simulink model "two_dof_arm_with_lqr_with_simscape"  (R2023a)
settings: Solver=FixedStepAuto  StartTime=0.0  StopTime=5  FixedStep=0.001  RelTol=1e-3
InitFcn:
  | two_link_planar_manipulator_sim
values from neighbouring files (symbols this model uses):
  g = [0 -9.81 0]    [two_link_planar_manipulator_sim.m]
  K = lqr(A,B,Q,R)    [two_link_planar_manipulator_sim.m]
  l = [0.25 0.25]    [two_link_planar_manipulator_sim.m]
  m = [1 1]    [two_link_planar_manipulator_sim.m]
  offset_error = 0.0175    [two_link_planar_manipulator_sim.m]
  resolution = 2^12    (= 4096)    [two_link_planar_manipulator_sim.m]
  sample_time = 0.001    [two_link_planar_manipulator_sim.m]
  true_delay = floor(delay*10^-3/sample_time)+sample_time*10^3    [two_link_planar_manipulator_sim.m]
  w = [0.04 0.04]    [two_link_planar_manipulator_sim.m]
  without_actuator_dynamics = true    [two_link_planar_manipulator_sim.m]
  without_meas_uncertainty = false    [two_link_planar_manipulator_sim.m]
libraries: sm_lib x12, nesl_utility x7, spsFirstOrderFilterLib x2, simulink x2, robotmaniplib x1, robotcorelib x1
settings Model: Creator=Jordan  LastModifiedBy=ddominguezmoises

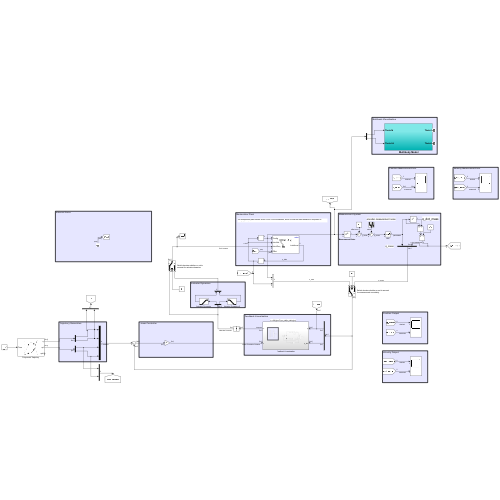
[thumbnail: Simulink's stored preview of the top-level diagram]
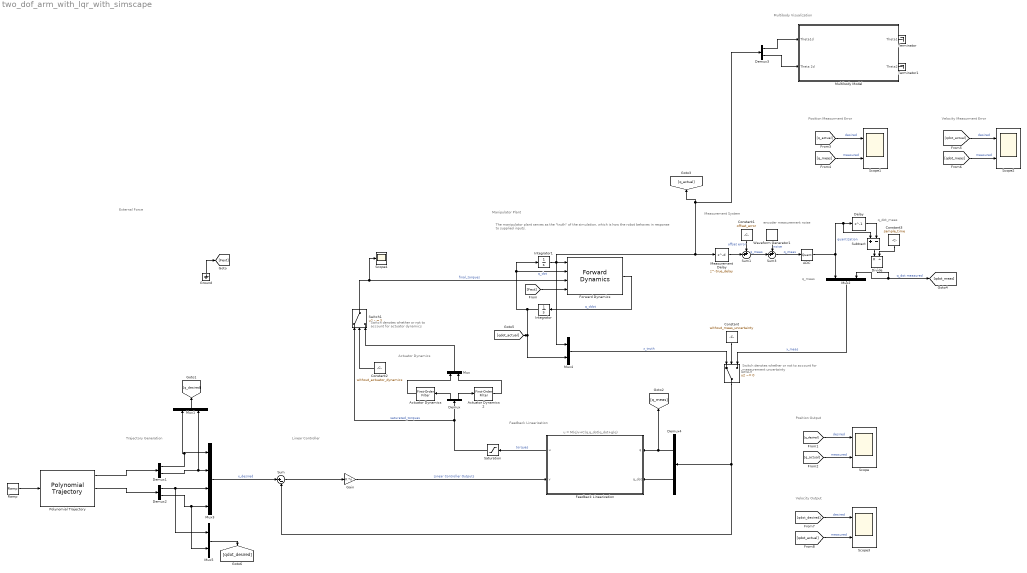
== system two_dof_arm_with_lqr_with_simscape ==
  note: Position Output
  note: Actuator Dynamics
  note: Switch denotes whether or not to account for actuator dynamics
  note: Switch denotes whether or not to account for measurement uncertainty
  note: u = M(q)v+C(q,q_dot)q_dot+g(q)
  note: Manipulator Plant
  note: The manipulator plant serves as the "truth" of the simulation, which is how the robot behaves in response to supplied inputs.
  note: Trajectory Generation
  note: Linear Controller
  note: Measurement System
  note: q_dot_meas
  note: encoder measurement noise
  note: q_meas
  note: Feedback Linearization
  note: External Force
  note: Position Measurment Error
  note: Velocity Measurment Error
  note: Velocity Output
  note: Multibody Visualization
  " Multibody Model" : Subsystem
  ADC : Quantizer  QuantizationInterval=2*pi/resolution  LinearizeAsGain=off
  Actuator Dynamics : spsFirstOrderFilterLib/First-Order Filter  FilterType=Lowpass  Tc=4.389e-4  Ts=0  Initialize=off  Vac_Init=[0, 0, 60]  Vdc_Init=0  PlotResponse=off  FreqRange="[0,  200,  1]"
  Actuator Dynamics 2 : spsFirstOrderFilterLib/First-Order Filter  FilterType=Lowpass  Tc=4.389e-4  Ts=0  Initialize=off  Vac_Init=[0, 0, 60]  Vdc_Init=0  PlotResponse=off  FreqRange="[0,  200,  1]"
  Constant : Constant  Value=without_meas_uncertainty
  Constant1 : Constant  Value=offset_error
  Constant2 : Constant  Value=without_actuator_dynamics
  Constant3 : Constant  Value=sample_time
  Delay : Delay  DelayLength=1
  Demux{,1..4} (5 alike) : Demux  Outputs=2
  Divide : Product  Inputs=*/
  Feedback Linearization : Subsystem
      settings: PortSchema="{\"entries\":[{\"content\":{\"sides\":[{\"content\":{\"connectorIds\":[\"In1\",\"In2\"]},\"type\":\"ConnectorPlacement.EquallySpacedRectSide\",\"uuid\":\"e20634ac-7282-4506-b427-a1989d27ee42\"},{\"content\":{\"connectorIds\":[\"Out1\",\"In3\"],\"side\":\"RIGHT\"},\"type\":\"ConnectorPlacement.EquallySpacedRectSide\",\"uuid\":\"ff8f2b23-ed86-4124-b979-83474755293e\"},{\"content\":{\"side\":\"TOP\"},\"type\":\"ConnectorPlacement.EquallySpacedRectSide\",\"uuid\":\"75dc970f-ba8d-4ce0-9b15-e79bd05d50ba\"}]},\"type\":\"ConnectorPlacement.EquallySpacedConnector\",\"uuid\":\"cd5a2392-675b-4624-9569-e6445bfb2136\"}],\"packageUris\":[\"http://schema.mathworks.com/mf0/Connector/R2020b\"],\"version\":\"1.0\"}"
  Forward Dynamics : robotmaniplib/Forward Dynamics  RigidBodyTree=robot  SimulateUsing=Interpreted execution
  Gain : Gain  Gain=K  Multiplication=Matrix(K*u)
  Ground : Ground
  Integrator : Integrator  InitialCondition=[0;0]
  Integrator1 : Integrator  InitialCondition=[0;0]
  Measurement Delay : Delay  DelayLength=true_delay
  Mux{,1..2,4..5} (5 alike) : Mux  Inputs=2
  Mux3 : Mux
  Polynomial Trajectory : robotcorelib/Polynomial Trajectory  WaypointSource=Internal  Waypoints=[ 0, 0, pi/2; 0, 0, pi/2]  TimePoints=[ 0, 1, 1.5]  TimeInterval=[ 1, 4 ]  Method=Cubic Polynomial  ParameterSource=Internal  VelocityBoundaryCondition=zeros( 2, 3 )  AccelerationBoundaryCondition=zeros( 2, 3 )  SimulateUsing=Interpreted execution
  Ramp : simulink/Sources/Ramp  slope=1  start=0  InitialOutput=0
  Saturation : Saturate  UpperLimit=150  LowerLimit=-150
  Scope{,1..3} (4 alike) : Scope  NumInputPorts=2
  Scope4 : Scope
  Subtract : Sum  Inputs=+-
  Sum : Sum  Inputs=|+-
  Sum1 : Sum  Inputs=++|
  Sum3 : Sum  Inputs=++|
  Switch : Switch  Criteria=u2 ~= 0  SaturateOnIntegerOverflow=off  InputSameDT=off
  Switch1 : Switch  Criteria=u2 ~= 0  SaturateOnIntegerOverflow=off  InputSameDT=off
  Terminator : Terminator
  Terminator1 : Terminator
  Waveform Generator1 : simulink/Sources/Waveform Generator  OutMin=[]  OutMax=[]  OutDataTypeStr=double  SelectedSignal=1  Signals=gaussian(mean,variance, seed)#gaussian(mean,variance, seed)  BlockNames=MultiportSwitch_510e73f99105412#MultiportSwitch_1249e3761ae8455  SampleTime=0.1
  wires:
  Integrator/1 -> [qdot_actual], Mux4/2, Integrator1/1, Forward Dynamics/2  "q_dot"
  Forward Dynamics/1 -> Integrator/1  "q_ddot"
  Delay/1 -> Subtract/2
  Sum3/1 -> ADC/1  "q_meas"
  Waveform Generator1/1 -> Sum3/1  "noise"
  Feedback Linearization/1(u) -> Saturation/1  "torques"
  Demux4/1 -> Feedback Linearization/1(q), [q_meas]
  Demux4/2 -> Feedback Linearization/2(q_dot)
  Gain/1 -> Feedback Linearization/3(v)  "Linear Controller Outputs"
  Ground/1 -> [Fext]
  [Fext] -> Forward Dynamics/4
  Sum1/1 -> Sum3/2  "q_meas"
  Constant1/1 -> Sum1/1  "offset error"
  Measurement Delay/1 -> Sum1/2
  ADC/1 -> Subtract/1, Delay/1, Mux2/1  "quantization"
  Demux/2 -> Actuator Dynamics 2/1
  Demux/1 -> Actuator Dynamics/1
  Actuator Dynamics/1 -> Mux/1
  Actuator Dynamics 2/1 -> Mux/2
  Mux1/1 -> [q_desired]
  Mux3/1 -> Sum/1  "x_desired"
  Sum/1 -> Gain/1
  Mux4/1 -> Switch/1  "x_truth"
  Mux2/1 -> Switch/3  "x_meas"
  Constant/1 -> Switch/2
  Switch/1 -> Demux4/1, Sum/2
  Switch1/1 -> Scope4/1, Forward Dynamics/3  "final_torques"
  Constant2/1 -> Switch1/2
  [q_desired] -> Scope/1  "desired"
  [q_actual] -> Scope/2  "measured"
  [q_actual] -> Scope1/1  "desired"
  [q_meas] -> Scope1/2  "measured"
  Subtract/1 -> Divide/1
  Constant3/1 -> Divide/2
  Divide/1 -> [qdot_meas], Mux2/2  "q_dot measured"
  [qdot_meas] -> Scope2/2  "measured"
  [qdot_actual] -> Scope2/1  "desired"
  [qdot_actual] -> Scope3/2  "measured"
  [qdot_desired] -> Scope3/1  "desired"
  Mux5/1 -> [qdot_desired]
  Mux/1 -> Switch1/3
  Ramp/1 -> Polynomial Trajectory/1
  Polynomial Trajectory/1 -> Demux1/1
  Demux1/1 -> Mux1/1, Mux3/1
  Demux1/2 -> Mux1/2, Mux3/2
  Polynomial Trajectory/2 -> Demux2/1
  Demux2/1 -> Mux5/1, Mux3/3
  Demux2/2 -> Mux5/2, Mux3/4
  Saturation/1 -> Demux/1, Switch1/1  "saturated_torques"
  " Multibody Model"/1(Theta1) -> Terminator/1
  " Multibody Model"/2(Theta2) -> Terminator1/1
  Demux3/2 -> " Multibody Model"/2(Theta 2d)
  Demux3/1 -> " Multibody Model"/1(Theta1d)
  Integrator1/1 -> Forward Dynamics/1, Mux4/1, Measurement Delay/1, Demux3/1, [q_actual]

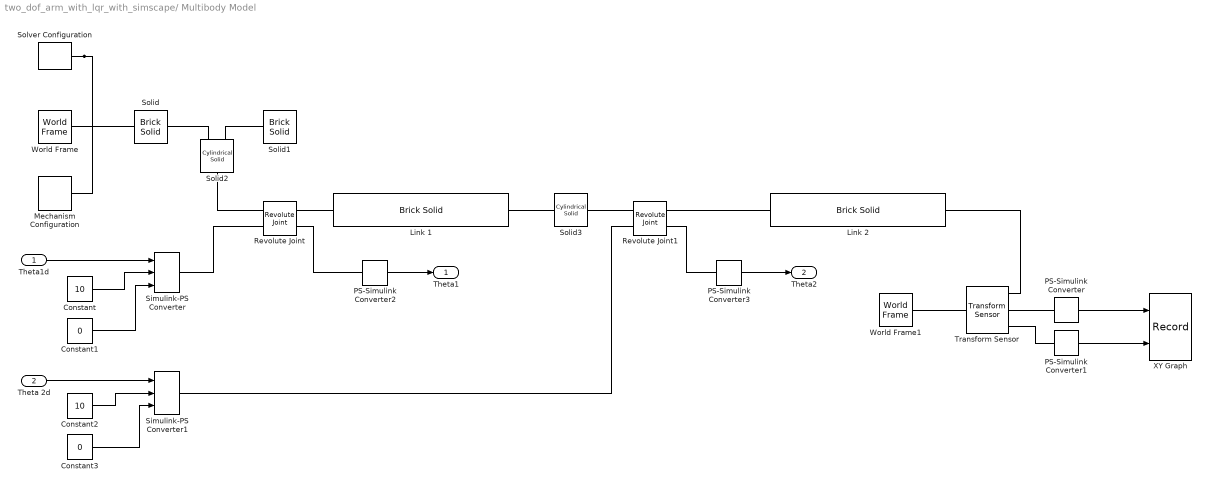
== system two_dof_arm_with_lqr_with_simscape/ Multibody Model ==
  Theta1d : Inport
  Theta 2d : Inport  Port=2
  Constant : Constant  Value=10
  Constant1 : Constant  Value=0
  Constant2 : Constant  Value=10
  Constant3 : Constant  Value=0
  Link 1 : sm_lib/Body Elements/Brick Solid  GraphicAmbientColor=[0.15 0.15 0.15 1.0]  BasedOnType=Density  BrickDimensions=[100 15 5]  BrickDimensionsUnits=cm  CenterOfMass=[0 0 0]  CenterOfMassUnits=m  GraphicDiffuseColor=[1.0 0.4 0.4]  Density=1000  DensityUnits=kg/m^3  DoExposeReferenceFrame=off  GraphicEmissiveColor=[0.0 0.0 0.0 1.0]  ExportEntireGeometry=off  SerializedFrames=<Frames><Frame><Id>Frame1</Id><Value><Name>L</Name><Origin><Source>GeometricFeature</Source><FeatureName>-x surface</FeatureName></Origin><PrimaryAxis><DefinedDirection>+Z</DefinedDirection><Source>ReferenceFrame</Source><SourceDirection>+Z</SourceDirection><FeatureName></FeatureName></PrimaryAxis><SecondaryAxis><DefinedDirection>+X</DefinedDirection><Source>ReferenceFrame</Source><SourceDirection>+X</SourceDirection><FeatureName></FeatureName></SecondaryAxis></Value></Frame><Frame><Id>Frame2</Id><Value><Name>R</Name><Origin><Source>GeometricFeature</Source><FeatureName>+x surface</FeatureName></Origin><PrimaryAxis><DefinedDirection>+Z</DefinedDirection><Source>ReferenceFrame</Source><SourceDirection>+Z</SourceDirection><FeatureName></FeatureName></PrimaryAxis><SecondaryAxis><DefinedDirection>+X</DefinedDirection><Source>ReferenceFrame</Source><SourceDirection>+X</SourceDirection><FeatureName></FeatureName></SecondaryAxis></Value></Frame></Frames>  MarkerShape=Sphere  MarkerSize=10  GraphicType=FromGeometry  InertiaType=CalculateFromGeometry  Mass=1  MassUnits=kg  MomentsOfInertia=[1 1 1]  MomentsOfInertiaUnits=kg*m^2  GraphicOpacity=1.0  ProductsOfInertia=[1 1 1]  ProductsOfInertiaUnits=kg*m^2  GraphicShininess=75  GraphicSpecularColor=[0.5 0.5 0.5 1.0]  GraphicVisPropType=SimpleVisualProperties
  Link 2 : sm_lib/Body Elements/Brick Solid  GraphicAmbientColor=[0.15 0.15 0.15 1.0]  BasedOnType=Density  BrickDimensions=[100 15 5]  BrickDimensionsUnits=cm  CenterOfMass=[0 0 0]  CenterOfMassUnits=m  GraphicDiffuseColor=[0.0 0.4 0.0]  Density=1000  DensityUnits=kg/m^3  DoExposeReferenceFrame=off  GraphicEmissiveColor=[0.0 0.0 0.0 1.0]  ExportEntireGeometry=off  SerializedFrames=<Frames><Frame><Id>Frame1</Id><Value><Name>L</Name><Origin><Source>GeometricFeature</Source><FeatureName>-x surface</FeatureName></Origin><PrimaryAxis><DefinedDirection>+Z</DefinedDirection><Source>ReferenceFrame</Source><SourceDirection>+Z</SourceDirection><FeatureName></FeatureName></PrimaryAxis><SecondaryAxis><DefinedDirection>+X</DefinedDirection><Source>ReferenceFrame</Source><SourceDirection>+X</SourceDirection><FeatureName></FeatureName></SecondaryAxis></Value></Frame><Frame><Id>Frame2</Id><Value><Name>R</Name><Origin><Source>GeometricFeature</Source><FeatureName>+x surface</FeatureName></Origin><PrimaryAxis><DefinedDirection>+Z</DefinedDirection><Source>ReferenceFrame</Source><SourceDirection>+Z</SourceDirection><FeatureName></FeatureName></PrimaryAxis><SecondaryAxis><DefinedDirection>+X</DefinedDirection><Source>ReferenceFrame</Source><SourceDirection>+X</SourceDirection><FeatureName></FeatureName></SecondaryAxis></Value></Frame></Frames>  MarkerShape=Sphere  MarkerSize=10  GraphicType=FromGeometry  InertiaType=CalculateFromGeometry  Mass=1  MassUnits=kg  MomentsOfInertia=[1 1 1]  MomentsOfInertiaUnits=kg*m^2  GraphicOpacity=1.0  ProductsOfInertia=[1 1 1]  ProductsOfInertiaUnits=kg*m^2  GraphicShininess=75  GraphicSpecularColor=[0.5 0.5 0.5 1.0]  GraphicVisPropType=SimpleVisualProperties
  Mechanism Configuration : sm_lib/Utilities/Mechanism Configuration  UniformGravity=Constant  GravityVector=[0 -9.80665 0]  GravityVectorUnits=m/s^2  LinearizationDelta=0.001  JointModeTransitionNonlinearIterations=2
  PS-Simulink Converter{,1..3} (4 alike) : nesl_utility/PS-Simulink Converter  PhysicalDomain=network_engine_domain  SubClassName=ps_output  LeftPortType=input  RightPortType=output  PseudoPeriodic=off  Frequencies=[]  VectorFormat=1-D array  Unit=1  AffineConversion=off
  Revolute Joint : sm_lib/Joints/Revolute Joint  JointMode=Normal  SenseConstraintForce=off  SenseConstraintForceX=off  SenseConstraintForceY=off  SenseConstraintForceZ=off  SenseConstraintTorque=off  SenseConstraintTorqueX=off  SenseConstraintTorqueY=off  SenseConstraintTorqueZ=off  SenseTotalForce=off  SenseTotalForceX=off  SenseTotalForceY=off  SenseTotalForceZ=off  SenseTotalTorque=off  SenseTotalTorqueX=off  SenseTotalTorqueY=off  SenseTotalTorqueZ=off  CompositeWrenchDir=FollowerOnBase  CompositeWrenchFrame=BaseFrame  EquilibriumPosition=0  EquilibriumPositionUnits=deg  SpringStiffness=0  SpringStiffnessUnits=N*m/deg  DampingCoefficient=0  DampingCoefficientUnits=N*m/(deg/s)  TorqueActuationMode=ComputedTorque  MotionActuationMode=InputMotion  SensePosition=on  SenseVelocity=off  SenseAcceleration=off  SenseTorqueForce=off  SenseLowerLimitTorqueForce=off  SenseUpperLimitTorqueForce=off  LowerLimitSpecify=off  LowerLimitBound=-90  LowerLimitBoundUnits=deg  LowerLimitStiffness=1e4  LowerLimitStiffnessUnits=N*m/deg  LowerLimitDamping=10  LowerLimitDampingUnits=N*m/(deg/s)  LowerLimitTransitionRegionWidth=0.1  LowerLimitTransitionRegionWidthUnits=deg  UpperLimitSpecify=off  UpperLimitBound=90  UpperLimitBoundUnits=deg  UpperLimitStiffness=1e4  UpperLimitStiffnessUnits=N*m/deg  UpperLimitDamping=10  UpperLimitDampingUnits=N*m/(deg/s)  UpperLimitTransitionRegionWidth=0.1  UpperLimitTransitionRegionWidthUnits=deg  PositionTargetSpecify=off  PositionTargetPriority=High  PositionTargetValue=0  PositionTargetValueUnits=deg  VelocityTargetSpecify=off  VelocityTargetPriority=High  VelocityTargetValue=0  VelocityTargetValueUnits=deg/s
  Revolute Joint1 : sm_lib/Joints/Revolute Joint  JointMode=Normal  SenseConstraintForce=off  SenseConstraintForceX=off  SenseConstraintForceY=off  SenseConstraintForceZ=off  SenseConstraintTorque=off  SenseConstraintTorqueX=off  SenseConstraintTorqueY=off  SenseConstraintTorqueZ=off  SenseTotalForce=off  SenseTotalForceX=off  SenseTotalForceY=off  SenseTotalForceZ=off  SenseTotalTorque=off  SenseTotalTorqueX=off  SenseTotalTorqueY=off  SenseTotalTorqueZ=off  CompositeWrenchDir=FollowerOnBase  CompositeWrenchFrame=BaseFrame  EquilibriumPosition=0  EquilibriumPositionUnits=deg  SpringStiffness=0  SpringStiffnessUnits=N*m/deg  DampingCoefficient=0  DampingCoefficientUnits=N*m/(deg/s)  TorqueActuationMode=ComputedTorque  MotionActuationMode=InputMotion  SensePosition=on  SenseVelocity=off  SenseAcceleration=off  SenseTorqueForce=off  SenseLowerLimitTorqueForce=off  SenseUpperLimitTorqueForce=off  LowerLimitSpecify=off  LowerLimitBound=-90  LowerLimitBoundUnits=deg  LowerLimitStiffness=1e4  LowerLimitStiffnessUnits=N*m/deg  LowerLimitDamping=10  LowerLimitDampingUnits=N*m/(deg/s)  LowerLimitTransitionRegionWidth=0.1  LowerLimitTransitionRegionWidthUnits=deg  UpperLimitSpecify=off  UpperLimitBound=90  UpperLimitBoundUnits=deg  UpperLimitStiffness=1e4  UpperLimitStiffnessUnits=N*m/deg  UpperLimitDamping=10  UpperLimitDampingUnits=N*m/(deg/s)  UpperLimitTransitionRegionWidth=0.1  UpperLimitTransitionRegionWidthUnits=deg  PositionTargetSpecify=off  PositionTargetPriority=High  PositionTargetValue=0  PositionTargetValueUnits=deg  VelocityTargetSpecify=off  VelocityTargetPriority=High  VelocityTargetValue=0  VelocityTargetValueUnits=deg/s
  Simulink-PS Converter : nesl_utility/Simulink-PS Converter  PhysicalDomain=network_engine_domain  SubClassName=ps_input  LeftPortType=input  RightPortType=output  PseudoPeriodic=off  Frequencies=[]  NoiseDistribution=none  NoiseParameters=[]  Unit=1  AffineConversion=off  FilteringAndDerivatives=provide  SimscapeFilterOrder=1  InputFilterTimeConstant=0.001  UdotUserProvided=2
  Simulink-PS Converter1 : nesl_utility/Simulink-PS Converter  PhysicalDomain=network_engine_domain  SubClassName=ps_input  LeftPortType=input  RightPortType=output  PseudoPeriodic=off  Frequencies=[]  NoiseDistribution=none  NoiseParameters=[]  Unit=1  AffineConversion=off  FilteringAndDerivatives=provide  SimscapeFilterOrder=1  InputFilterTimeConstant=0.001  UdotUserProvided=2
  Solid : sm_lib/Body Elements/Brick Solid  GraphicAmbientColor=[0.15 0.15 0.15 1.0]  BasedOnType=Density  BrickDimensions=[15 15 5]  BrickDimensionsUnits=cm  CenterOfMass=[0 0 0]  CenterOfMassUnits=m  GraphicDiffuseColor=[0.0 0.0 0.6]  Density=1000  DensityUnits=kg/m^3  DoExposeReferenceFrame=on  GraphicEmissiveColor=[0.0 0.0 0.0 1.0]  ExportEntireGeometry=off  SerializedFrames=<Frames><Frame><Id>Frame1</Id><Value><Name>F</Name><Origin><Source>GeometricFeature</Source><FeatureName>-z surface</FeatureName></Origin><PrimaryAxis><DefinedDirection>+Z</DefinedDirection><Source>ReferenceFrame</Source><SourceDirection>+Z</SourceDirection><FeatureName></FeatureName></PrimaryAxis><SecondaryAxis><DefinedDirection>+X</DefinedDirection><Source>ReferenceFrame</Source><SourceDirection>+X</SourceDirection><FeatureName></FeatureName></SecondaryAxis></Value></Frame></Frames>  MarkerShape=Sphere  MarkerSize=10  GraphicType=FromGeometry  InertiaType=CalculateFromGeometry  Mass=1  MassUnits=kg  MomentsOfInertia=[1 1 1]  MomentsOfInertiaUnits=kg*m^2  GraphicOpacity=1.0  ProductsOfInertia=[1 1 1]  ProductsOfInertiaUnits=kg*m^2  GraphicShininess=75  GraphicSpecularColor=[0.5 0.5 0.5 1.0]  GraphicVisPropType=SimpleVisualProperties
  Solid1 : sm_lib/Body Elements/Brick Solid  GraphicAmbientColor=[0.15 0.15 0.15 1.0]  BasedOnType=Density  BrickDimensions=[15 15 5]  BrickDimensionsUnits=cm  CenterOfMass=[0 0 0]  CenterOfMassUnits=m  GraphicDiffuseColor=[0.0 0.0 0.6]  Density=1000  DensityUnits=kg/m^3  DoExposeReferenceFrame=off  GraphicEmissiveColor=[0.0 0.0 0.0 1.0]  ExportEntireGeometry=off  SerializedFrames=<Frames><Frame><Id>Frame1</Id><Value><Name>F</Name><Origin><Source>GeometricFeature</Source><FeatureName>+z surface</FeatureName></Origin><PrimaryAxis><DefinedDirection>+Z</DefinedDirection><Source>ReferenceFrame</Source><SourceDirection>+Z</SourceDirection><FeatureName></FeatureName></PrimaryAxis><SecondaryAxis><DefinedDirection>+X</DefinedDirection><Source>ReferenceFrame</Source><SourceDirection>+X</SourceDirection><FeatureName></FeatureName></SecondaryAxis></Value></Frame></Frames>  MarkerShape=Sphere  MarkerSize=10  GraphicType=FromGeometry  InertiaType=CalculateFromGeometry  Mass=1  MassUnits=kg  MomentsOfInertia=[1 1 1]  MomentsOfInertiaUnits=kg*m^2  GraphicOpacity=1.0  ProductsOfInertia=[1 1 1]  ProductsOfInertiaUnits=kg*m^2  GraphicShininess=75  GraphicSpecularColor=[0.5 0.5 0.5 1.0]  GraphicVisPropType=SimpleVisualProperties
  Solid2 : sm_lib/Body Elements/Cylindrical Solid  GraphicAmbientColor=[0.15 0.15 0.15 1.0]  BasedOnType=Density  CenterOfMass=[0 0 0]  CenterOfMassUnits=m  GraphicDiffuseColor=[0.0 0.0 0.6]  CylinderLength=6  CylinderLengthUnits=cm  CylinderRadius=5  CylinderRadiusUnits=cm  Density=1000  DensityUnits=kg/m^3  DoExposeReferenceFrame=on  GraphicEmissiveColor=[0.0 0.0 0.0 1.0]  ExportEntireGeometry=off  SerializedFrames=<Frames><Frame><Id>Frame1</Id><Value><Name>L</Name><Origin><Source>GeometricFeature</Source><FeatureName>top surface</FeatureName></Origin><PrimaryAxis><DefinedDirection>+Z</DefinedDirection><Source>ReferenceFrame</Source><SourceDirection>+Z</SourceDirection><FeatureName></FeatureName></PrimaryAxis><SecondaryAxis><DefinedDirection>+X</DefinedDirection><Source>ReferenceFrame</Source><SourceDirection>+X</SourceDirection><FeatureName></FeatureName></SecondaryAxis></Value></Frame><Frame><Id>Frame2</Id><Value><Name>R</Name><Origin><Source>GeometricFeature</Source><FeatureName>bottom surface</FeatureName></Origin><PrimaryAxis><DefinedDirection>+Z</DefinedDirection><Source>ReferenceFrame</Source><SourceDirection>+Z</SourceDirection><FeatureName></FeatureName></PrimaryAxis><SecondaryAxis><DefinedDirection>+X</DefinedDirection><Source>ReferenceFrame</Source><SourceDirection>+X</SourceDirection><FeatureName></FeatureName></SecondaryAxis></Value></Frame></Frames>  MarkerShape=Sphere  MarkerSize=10  GraphicType=FromGeometry  InertiaType=CalculateFromGeometry  Mass=1  MassUnits=kg  MomentsOfInertia=[1 1 1]  MomentsOfInertiaUnits=kg*m^2  GraphicOpacity=1.0  ProductsOfInertia=[1 1 1]  ProductsOfInertiaUnits=kg*m^2  GraphicShininess=75  GraphicSpecularColor=[0.5 0.5 0.5 1.0]  GraphicVisPropType=SimpleVisualProperties
  Solid3 : sm_lib/Body Elements/Cylindrical Solid  GraphicAmbientColor=[0.15 0.15 0.15 1.0]  BasedOnType=Density  CenterOfMass=[0 0 0]  CenterOfMassUnits=m  GraphicDiffuseColor=[0.8 0.0 0.0]  CylinderLength=6  CylinderLengthUnits=cm  CylinderRadius=5  CylinderRadiusUnits=cm  Density=1000  DensityUnits=kg/m^3  DoExposeReferenceFrame=off  GraphicEmissiveColor=[0.0 0.0 0.0 1.0]  ExportEntireGeometry=off  SerializedFrames=<Frames><Frame><Id>Frame1</Id><Value><Name>L</Name><Origin><Source>GeometricFeature</Source><FeatureName>top surface</FeatureName></Origin><PrimaryAxis><DefinedDirection>+Z</DefinedDirection><Source>ReferenceFrame</Source><SourceDirection>+Z</SourceDirection><FeatureName></FeatureName></PrimaryAxis><SecondaryAxis><DefinedDirection>+X</DefinedDirection><Source>ReferenceFrame</Source><SourceDirection>+X</SourceDirection><FeatureName></FeatureName></SecondaryAxis></Value></Frame><Frame><Id>Frame2</Id><Value><Name>R</Name><Origin><Source>GeometricFeature</Source><FeatureName>bottom surface</FeatureName></Origin><PrimaryAxis><DefinedDirection>+Z</DefinedDirection><Source>ReferenceFrame</Source><SourceDirection>+Z</SourceDirection><FeatureName></FeatureName></PrimaryAxis><SecondaryAxis><DefinedDirection>+X</DefinedDirection><Source>ReferenceFrame</Source><SourceDirection>+X</SourceDirection><FeatureName></FeatureName></SecondaryAxis></Value></Frame></Frames>  MarkerShape=Sphere  MarkerSize=10  GraphicType=FromGeometry  InertiaType=CalculateFromGeometry  Mass=1  MassUnits=kg  MomentsOfInertia=[1 1 1]  MomentsOfInertiaUnits=kg*m^2  GraphicOpacity=1.0  ProductsOfInertia=[1 1 1]  ProductsOfInertiaUnits=kg*m^2  GraphicShininess=75  GraphicSpecularColor=[0.5 0.5 0.5 1.0]  GraphicVisPropType=SimpleVisualProperties
  Solver Configuration : nesl_utility/Solver Configuration  PhysicalDomain=network_engine_domain  SubClassName=solver  LeftPortType=input  RightPortType=generic  Tones=[]  Harmonics=[]  SimulateNoise=off  Profile=off  UseLocalSampling=off  EnableSwitchedLinearOptims=on  FrequencyDomain=off  UseCCode=off  RelTol=0.001  AbsTol=1e-06  MinStep=1e-09  ToWorkspace=off  RevertToSquareIcSolve=off  NumHomotopyIterations=100  PhasorMode=off  PhasorModeNumHarmonics=1  ConsistencySolver=NEWTON_FTOL  IndexReductionMethod=DerivativeReplacement  DoDC=off  ResidualTolerance=1e-09  ConsistencyTolSource=GLOBAL  ConsistencyAbsTol=0.001  ConsistencyRelTol=0.001  ConsistencyTolFactor=0.001  UseLocalSolver=off  LocalSolverChoice=NE_BACKWARD_EULER_ADVANCER  ResolveIndetEquations=on  FunctionEvalNumThread=1  LocalSolverSampleTime=0.001  DoFixedCost=off  MaxNonlinIter=3  MaxModeIter=2  ComputeImpulses=off  ImpulseIterations=2  LinearAlgebra=Sparse  LinearAlgebraNumThread=0  EquationFormulation=NE_TIME_EF  DelaysMemoryBudget=1024  AutomaticFiltering=on  FilteringTimeConstant=0.001  PartitionStorageMethod=AS_NEEDED  PartitionMemoryBudget=1024  PartitionMethod=FAST
  Transform Sensor : sm_lib/Frames and Transforms/Transform Sensor  MeasurementFrame=World  RotationSequence=XYX  SenseAngle=off  SenseAxis=off  SenseQ=off  SenseR=off  SenseRotationSequence=off  SenseOmegaX=off  SenseOmegaY=off  SenseOmegaZ=off  SenseQDot=off  SenseRDot=off  SenseRotationSequenceDot=off  SenseAlphaX=off  SenseAlphaY=off  SenseAlphaZ=off  SenseQDDot=off  SenseRDDot=off  SenseX=on  SenseY=on  SenseZ=off  SenseRad=off  SenseAzim=off  SenseDist=off  SenseInc=off  SenseXDot=off  SenseYDot=off  SenseZDot=off  SenseRadDot=off  SenseAzimDot=off  SenseDistDot=off  SenseIncDot=off  SenseXDDot=off  SenseYDDot=off  SenseZDDot=off  SenseRadDDot=off  SenseAzimDDot=off  SenseDistDDot=off  SenseIncDDot=off
  World Frame : sm_lib/Frames and Transforms/World Frame
  World Frame1 : sm_lib/Frames and Transforms/World Frame
  XY Graph : Record  FileSettingsInternal="{\"entries\":[{\"content\":{\"excelSettings\":{\"content\":{},\"type\":\"Streamout.ExcelSettings\"}},\"type\":\"Streamout.FileSettingStorage\",\"uuid\":\"9ef0b3cf-b923-49fd-8610-193f2f58b0c9\"}],\"packageUris\":[\"http://schema.mathworks.com/mf0/streamout_blocks/R2020a\"],\"version\":\"1.0\"}"  Layout=[1 1]  SignalsInternal="{\"entries\":[{\"content\":{\"signals\":[{\"content\":{\"blockPath\":[\"two_dof_arm_with_lqr_with_simscape/ Multibody Model/XY Graph\"],\"dimensions\":[1],\"domain\":\"two_dof_arm_with_lqr_with_simscape/ Multibody Model/XY Graph\",\"lineColor\":\"#a2142f\",\"port\":1,\"sid\":[\"\"],\"signalID\":36,\"signalName\":\"PS-Simulink\\nConverter\"},\"type\":\"RecordBlkView.Signal\",\"uuid\":\"e07cb7e0-df82-4729-932e-b47a9a5ad0b3\"},{\"content\":{\"blockPath\":[\"two_dof_arm_with_lqr_with_simscape/ Multibody Model/XY Graph\"],\"dimensions\":[1],\"domain\":\"two_dof_arm_with_lqr_with_simscape/ Multibody Model/XY Graph\",\"lineColor\":\"#139fff\",\"port\":2,\"sid\":[\"\"],\"signalID\":41,\"signalName\":\"PS-Simulink\\nConverter1\"},\"type\":\"RecordBlkView.Signal\",\"uuid\":\"985cc778-3e0b-45ef-a594-7c9f007809c4\"}]},\"type\":\"RecordBlkView.InputSignals\",\"uuid\":\"fcb45d65-4978-4641-ab11-c30ee1f1961b\"}],\"packageUris\":[\"http://schema.mathworks.com/mf0/streamout_blocks/R2020a\"],\"version\":\"1.0\"}"  VisualizationBindings="{\"xyplotplugin\":{\"info\":[{\"series\":[],\"subplotID\":1}]}}"  CompatibilityTag=XY  st=-1
  Theta1 : Outport  VectorParamsAs1DForOutWhenUnconnected=off
  Theta2 : Outport  Port=2  VectorParamsAs1DForOutWhenUnconnected=off
  wires:
  PS-Simulink Converter/1 -> XY Graph/1
  Constant/1 -> Simulink-PS Converter/2
  Theta 2d/1 -> Simulink-PS Converter1/1
  PS-Simulink Converter1/1 -> XY Graph/2
  Theta1d/1 -> Simulink-PS Converter/1
  Constant1/1 -> Simulink-PS Converter/3
  PS-Simulink Converter2/1 -> Theta1/1
  Constant3/1 -> Simulink-PS Converter1/3
  Constant2/1 -> Simulink-PS Converter1/2
  PS-Simulink Converter3/1 -> Theta2/1
  connections:
  Link 2/LConn1 -- Revolute Joint1/RConn1
  Revolute Joint1/LConn1 -- Solid3/RConn1
  PS-Simulink Converter3/LConn1 -- Revolute Joint1/RConn2
  PS-Simulink Converter/LConn1 -- Transform Sensor/RConn2
  Transform Sensor/RConn3 -- PS-Simulink Converter1/LConn1
  Solver Configuration/RConn1 -- Solid/RConn1 -- Mechanism Configuration/RConn1 -- World Frame/RConn1
  Simulink-PS Converter1/RConn1 -- Revolute Joint1/LConn2
  Simulink-PS Converter/RConn1 -- Revolute Joint/LConn2
  PS-Simulink Converter2/LConn1 -- Revolute Joint/RConn2
  Revolute Joint/LConn1 -- Solid2/RConn1
  Solid2/LConn2 -- Solid1/LConn1
  Solid2/LConn1 -- Solid/LConn1
  Revolute Joint/RConn1 -- Link 1/LConn1
  Solid3/LConn1 -- Link 1/RConn1
  World Frame1/RConn1 -- Transform Sensor/LConn1
  Transform Sensor/RConn1 -- Link 2/RConn1

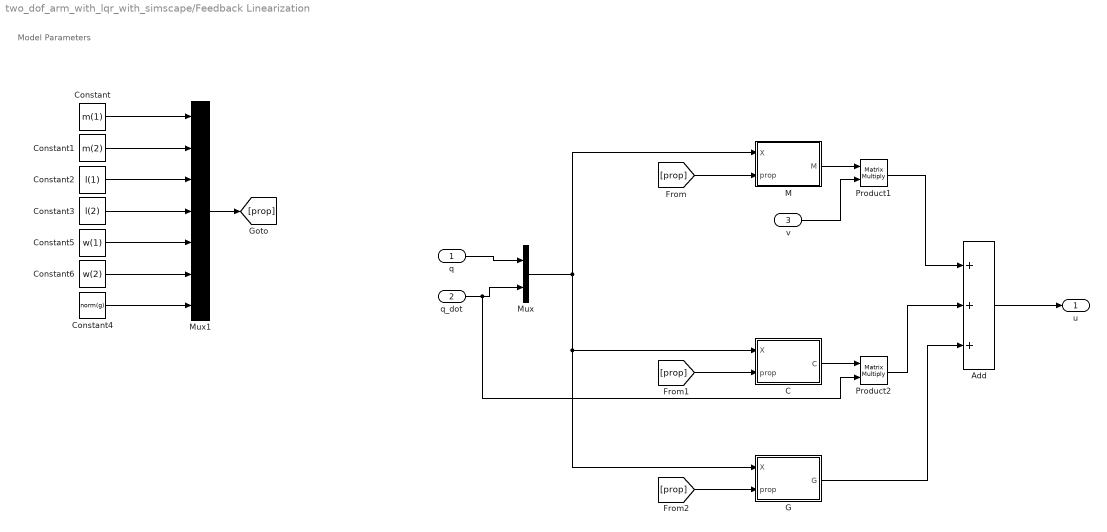
== system two_dof_arm_with_lqr_with_simscape/Feedback Linearization ==
  note: Model Parameters
  q : Inport  PortDimensions=[2 1]
  q_dot : Inport  Port=2  PortDimensions=[2 1]
  v : Inport  Port=3  PortDimensions=[2 1]
  Add : Sum  Inputs=+++
  C : MATLAB Function  TreatAsAtomicUnit=on
  Constant : Constant  Value=m(1)
  Constant1 : Constant  Value=m(2)
  Constant2 : Constant  Value=l(1)
  Constant3 : Constant  Value=l(2)
  Constant4 : Constant  Value=norm(g)
  Constant5 : Constant  Value=w(1)
  Constant6 : Constant  Value=w(2)
  G : MATLAB Function  TreatAsAtomicUnit=on
  M : MATLAB Function  TreatAsAtomicUnit=on
  Mux : Mux  Inputs=2
  Mux1 : Mux  Inputs=7
  Product1 : Product  Multiplication=Matrix(*)
  Product2 : Product  Multiplication=Matrix(*)
  u : Outport  PortDimensions=[2 1]
  wires:
  Constant1/1 -> Mux1/2
  Constant4/1 -> Mux1/7
  Mux1/1 -> [prop]
  Constant/1 -> Mux1/1
  [prop] -> G/2(prop)
  Constant2/1 -> Mux1/3
  [prop] -> C/2(prop)
  Constant3/1 -> Mux1/4
  [prop] -> M/2(prop)
  Mux/1 -> M/1(X), G/1(X), C/1(X)
  q/1 -> Mux/1
  q_dot/1 -> Product2/2, Mux/2
  M/1(M) -> Product1/1
  v/1 -> Product1/2
  Product1/1 -> Add/1
  G/1(G) -> Add/3
  Add/1 -> u/1
  C/1(C) -> Product2/1
  Product2/1 -> Add/2
  Constant5/1 -> Mux1/5
  Constant6/1 -> Mux1/6

== matlab function two_dof_arm_with_lqr_with_simscape/Feedback Linearization/G ==
  data: X input; G output; prop input
function G = fcn(X,prop)
    m1 = prop(1);
    m2 = prop(2);
    l1 = prop(3);
    l2 = prop(4);
    g = prop(7);
    theta1 = X(1);
    theta2 = X(2);
    r1 = l1/2;
    r2 = l2/2;
    
    G1 = g*m2*(r2*cos(theta1+theta2)+l1*cos(theta1))+g*m1*r1*cos(theta1);
    G2 = g*m2*r2*cos(theta1+theta2);
    
    G = [G1;G2];

== matlab function two_dof_arm_with_lqr_with_simscape/Feedback Linearization/M ==
  data: X input; M output; prop input
function M = fcn(X,prop)
    m1 = prop(1);
    m2 = prop(2);
    l1 = prop(3);
    l2 = prop(4);
    w1 = prop(5);
    w2 = prop(6);
    r1 = l1/2;
    r2 = l2/2;
    theta1 = X(1);
    theta2 = X(2);
    Iz1 = 1/12*m1*(l1^2+w1^2);
    Iz2 = 1/12*m2*(l2^2+w2^2);
    
    M11 = m2*l1^2+2*m2*cos(theta2)*l1*r2+m1*r1^2+m2*r2^2+Iz1+Iz2;
    M12 = m2*r2^2+l1*m2*cos(theta2)*r2+Iz2;
    M21 = m2*r2^2+l1*m2*cos(theta2)*r2+Iz2;
    M22 = m2*r2^2+Iz2;
    
    M = [M11 M12; M21 M22];

== matlab function two_dof_arm_with_lqr_with_simscape/Feedback Linearization/C ==
  data: X input; C output; prop input
function C = fcn(X,prop)
    m2 = prop(2);
    l1 = prop(3);
    l2 = prop(4);
    r2 = l2/2;
    theta1 = X(1);
    theta2 = X(2);
    theta1_dot = X(3);
    theta2_dot = X(4);
    
    C11 = -l1*m2*theta2_dot*r2*sin(theta2);
    C12 = -l1*m2*r2*sin(theta2)*(theta1_dot+theta2_dot);
    C21 = l1*m2*theta1_dot*r2*sin(theta2);
    C22 = 0;
    
    C = [C11 C12;C21 C22];
